simulink model "pendulosimples"  (R2016a)
settings: Solver=ode113  StartTime=0.0  StopTime=25  RelTol=1e-6
settings Model: Creator=asus  LastModifiedBy=asus
settings SolverCC: ZeroCrossAlgorithm=Adaptive
settings DataIOCC: LimitDataPoints=on  SaveFormat=Array
settings HardwareCC: ProdBitPerPointer=32  ProdLargestAtomicFloat=None  ProdIntDivRoundTo=Undefined  ProdEndianess=Unspecified  ProdWordSize=32  ProdHWDeviceType=32-bit Generic
settings ModelReferenceCC: PropagateSignalLabelsOutOfModel=off
settings ConfigComp: CovModelRefEnable=Off

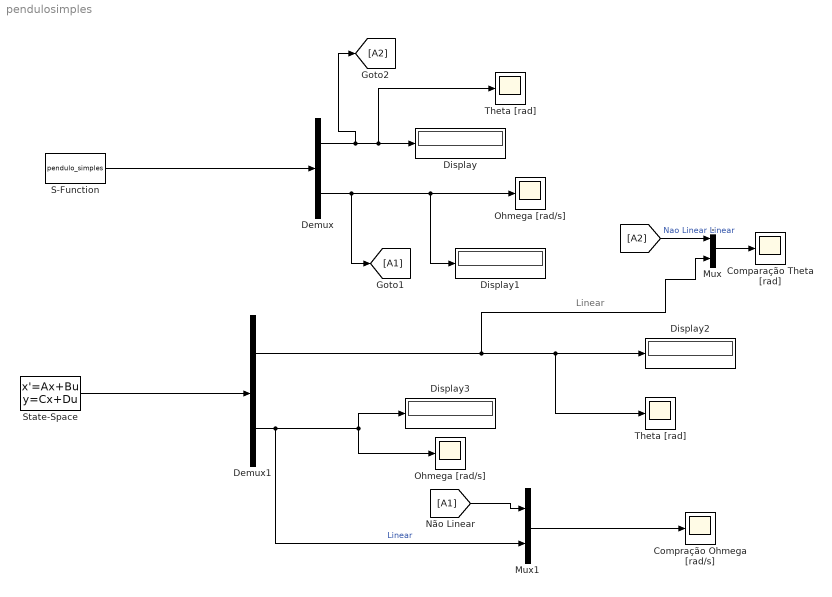
== system pendulosimples ==
  note: Linear
  "Comparação Theta [rad] " : Scope
  Compração Ohmega [rad/s] : Scope
  Demux : Demux  Outputs=2
  Demux1 : Demux  Outputs=2
  Display{,1..3} (4 alike) : Display
  Mux : Mux  Inputs=2
  Mux1 : Mux  Inputs=2
  Ohmega [rad/s] : Scope
  "Ohmega [rad/s]\t" : Scope
  S-Function : S-Function  FunctionName=pendulo_simples  Parameters=g, L  SFunctionDeploymentMode=off  EnableBusSupport=off  mask{g=9.81, L=0.5}
      mask prompts: g "Aceleracao gravidade [=] m/s^2"; L "Comprimento Corda[=] m"
  State-Space : StateSpace  A=[0 1; -19.62 0]  B=[0 0; 0 0]  C=[1 0;0 1]  D=[0 0;0 0]  X0=[pi/4; 0]
  Theta [rad] : Scope
  "Theta [rad] " : Scope
  wires:
  Demux/1 -> [A2], Theta [rad]/1, Display/1
  Demux/2 -> [A1], Display1/1, Ohmega [rad/s]/1
  S-Function/1 -> Demux/1
  State-Space/1 -> Demux1/1
  Demux1/2 -> Mux1/2, Display3/1, "Ohmega [rad/s]\t"/1  "Linear"
  Demux1/1 -> Mux/2, "Theta [rad] "/1, Display2/1
  [A1] -> Mux1/1
  Mux/1 -> "Comparação Theta [rad] "/1
  Mux1/1 -> Compração Ohmega [rad/s]/1
  [A2] -> Mux/1  "Nao Linear Linear"
